simulink model "Table_airbus_v1"  (R2021b)
settings: Solver=VariableStepAuto  StartTime=0.0  StopTime=20  MaxStep=0.01  RelTol=0.01
undefined symbols (not defined in the file): X, Y, Z
libraries: sm_lib x907, fl_lib x69, nesl_utility x53, sdl_lib x10, ee_lib x7, slpidlib x6, simulink x5, simulink_extras x4
(part 1 of 18)
settings Model: Creator=Marc  LastModifiedBy=mgarc
settings SolverCC: ZeroCrossAlgorithm=Adaptive  AlgebraicLoopSolver=TrustRegion
settings DebuggingCC: IgnoredZcDiagnostic=none  SFMachineParentedDataDiag=warning  ArithmeticOperatorsInVariantConditions=warning
settings SFSimCC: CustomCodeUndefinedFunction=UseInterfaceOnly
settings ExplorerConfigSet: InternalSimMechanicsExplorerSettings="<ExplorerConfiguration><canonicalview>default</canonicalview><AnimationSetting><BasePlaybackSpeed>1.0</BasePlaybackSpeed><PlaybackSpeedFactor>1.0</PlaybackSpeedFactor></AnimationSetting><TilePanel><TileInfo><Tiles Columns=\"2\" Count=\"4\" Rows=\"2\"><Column Weight=\"0.4997\"/><Column Weight=\"0.5003\"/><Row Weight=\"0.5\"/><Row Weight=\"0.5\"/><Tile Height=\"1\" Width=\"1\" X=\"0\" Y=\"0\"/><Tile Height=\"1\" Width=\"1\" X=\"0\" Y=\"1\"/><Tile Height=\"1\" Width=\"1\" X=\"1\" Y=\"0\"/><Tile Height=\"1\" Width=\"1\" X=\"1\" Y=\"1\"/></Tiles></TileInfo><SceneInfo><SceneViewer><BGColor><R>0.60000002384185791</R><G>0.60000002384185791</G><B>0.60000002384185791</B></BGColor><Camera><DoPerspective>off</DoPerspective><Position><X>-1.24933457614355525</X><Y>-1.70068668146841429</Y><Z>0.410584900495560123</Z></Position><Center><X>-1.24933457614355525</X><Y>1.97814830626974469e-08</Y><Z>0.410584900495560123</Z></Center><Up><X>0</X><Y>-0</Y><Z>1</Z></Up><ViewLimDist>1</ViewLimDist><YLim>0.703268185423852166</YLim><XLim>1.31924547195434561</XLim></Camera></SceneViewer><SceneViewer><BGColor><R>0.60000002384185791</R><G>0.60000002384185791</G><B>0.60000002384185791</B></BGColor><Camera><DoPerspective>off</DoPerspective><Position><X>-1.24933457614355525</X><Y>4.88032186884979069e-09</Y><Z>2.2537451526153367</Z></Position><Center><X>-1.24933457614355525</X><Y>4.88032186884979069e-09</Y><Z>0.410584900495560179</Z></Center><Up><X>0</X><Y>1</Y><Z>-0</Z></Up><ViewLimDist>1</ViewLimDist><YLim>0.703268185423852166</YLim><XLim>1.31924547195434561</XLim></Camera></SceneViewer><SceneViewer><BGColor><R>0.60000002384185791</R><G>0.60000002384185791</G><B>0.60000002384185791</B></BGColor><Camera><DoPerspective>off</DoPerspective><Position><X>0.330264279532568983</X><Y>4.88032181333863946e-09</Y><Z>0.410584900495559957</Z></Position><Center><X>-1.2493346738951725</X><Y>4.88032181333863946e-09</Y><Z>0.410584900495559957</Z></Center><Up><X>-0</X><Y>0</Y><Z>1</Z></Up><ViewLimDist>1</ViewLimDist><YLim>0.415614598393440282</YLim><XLim>0.780615709394705148</XLim></Camera></SceneViewer><SceneViewer><BGColor><R>0.60000002384185791</R><G>0.60000002384185791</G><B>0.60000002384185791</B></BGColor><Camera><DoPerspective>off</DoPerspective><Position><X>-0.231613369317086537</X><Y>-0.977872883847284546</Y><Z>1.37865497927362801</Z></Position><Center><X>-1.1321755767731061</X><Y>-0.0773106763912649875</Y><Z>0.47809277181760812</Z></Center><Up><X>-0.408248290463863073</X><Y>0.408248290463863073</Y><Z>0.816496580927726145</Z></Up><ViewLimDist>1</ViewLimDist><YLim>1.00376938045024877</YLim><XLim>1.88529986679414407</XLim></Camera></SceneViewer></SceneInfo></TilePanel><MechEditorPanel><Cameras/><GfxPanelCameraMap/><VideoCreator><PlaybackSpeedRatio>1.0</PlaybackSpeedRatio><FrameRate>30</FrameRate><VideoFormat>Motion JPEG AVI</VideoFormat><FrameSize>auto</FrameSize></VideoCreator></MechEditorPanel></ExplorerConfiguration>"

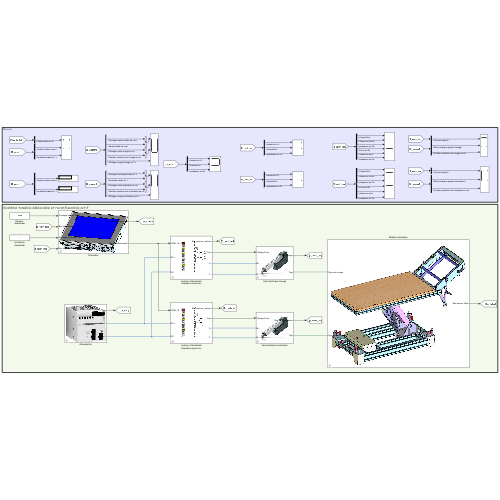
[thumbnail: Simulink's stored preview of the top-level diagram]
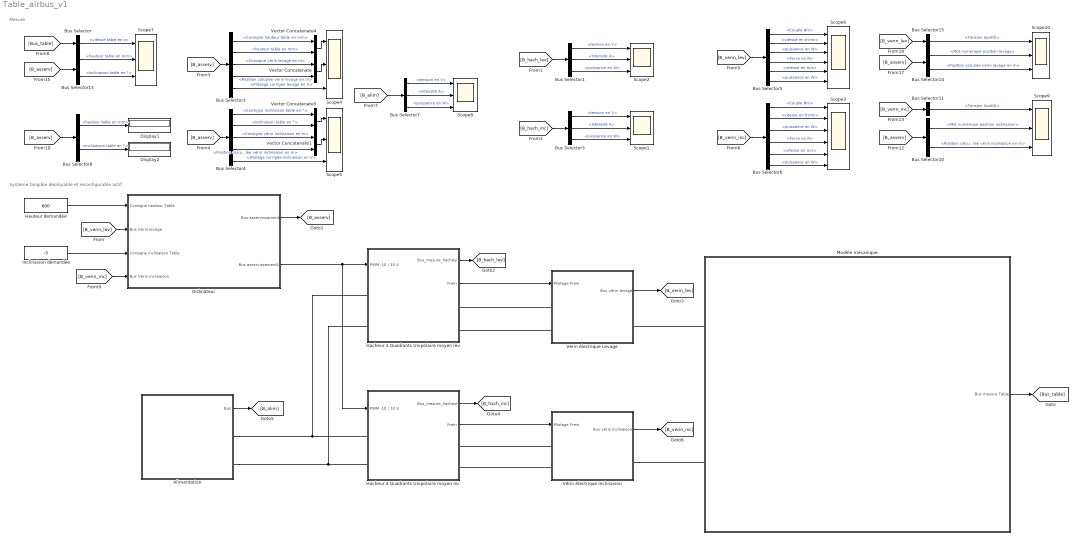
== system Table_airbus_v1 ==
  note: Mesure
  note: Système tangible déployable et reconfigurable actif
  Alimentation : Subsystem  mask{Ualim=36, Ralim=0.5}
      mask prompts: Ualim "Tension d'alimentation en V"; Ralim "Résistance interne alimentation en ohm"
      mask DialogControl ParameterGroupVar Prompt: Paramètres alimentation
      mask Display: image('alimentation.png')
  Bus Selector : BusSelector  OutputSignals=vitesse table en z
  Bus Selector1 : BusSelector  OutputSignals=tension en V,Intensité A,puissance en W
  Bus Selector10 : BusSelector  OutputSignals=Mot numérique position inclinaison,Position calculée vérin inclinaison en m
  Bus Selector11 : BusSelector  OutputSignals=Tension Upot(t)
  Bus Selector13 : BusSelector  OutputSignals=hauteur table en mm,Inclinaison table en °
  Bus Selector14 : BusSelector  OutputSignals=Mot numérique position levage,Position calculée vérin levage en m
  Bus Selector15 : BusSelector  OutputSignals=Tension Upot(t)
  Bus Selector2 : BusSelector  OutputSignals=Consigne hauteur table en mm,hauteur table en mm,Consigne vérin levage en m,Position calculée vérin levage en m,Pilotage corrigée levage en V
  Bus Selector3 : BusSelector  OutputSignals=tension en V,Intensité A,puissance en W
  Bus Selector4 : BusSelector  OutputSignals=Consigne inclinaison table en °,Inclinaison table en °,Consigne vérin inclinaison en m,Position calculée vérin inclinaison en m,Pilotage corrigée inclinaison en V
  Bus Selector5 : BusSelector  OutputSignals=Bus meca moteur.Couple Nm,Bus meca moteur.vitesse en tr/mn,Bus meca moteur.puissance en W,Bus vis écrou.Force en N,Bus vis écrou.vitesse en m/s,Bus vis écrou.puissance en W
  Bus Selector6 : BusSelector  OutputSignals=Bus meca moteur.Couple Nm,Bus meca moteur.vitesse en tr/mn,Bus meca moteur.puissance en W,Bus vis écrou.Force en N,Bus vis écrou.vitesse en m/s,Bus vis écrou.puissance en W
  Bus Selector7 : BusSelector  OutputSignals=tension en V,Intensité A,puissance en W
  Bus Selector8 : BusSelector  OutputSignals=hauteur table en mm,Inclinaison table en °
  Display1 : Display
  Display2 : Display
  Hacheur 4 Quadrants Unipolaire moyen Inc : Subsystem  mask{Rds=0.2, Rd=0.1, Vd=0.65, kpn=4, kin=1, kdn=0, Imax=8, Kpi=0.8, Kii=0, Kdi=0}
      mask prompts: Rds "Résistance drain source Mosfet en ohm"; Rd "Résistance diode source drain en ohm"; Vd "Tension de seuil diode source drain en volt"; kpn "Gain proportionnel"; kin "Gain intégral"; kdn "Gain dérivée"; Imax "Limitation d'intensité en A"; Kpi "Gain proportionnel"; Kii "Gain intégral"; Kdi "Gain dérivée"
      mask DialogControl ParameterGroupVar Prompt: Paramétrages carte d'axe
      mask DialogControl Container4 Prompt: Hacheur
      mask DialogControl Container5 Prompt: Régulation Vitesse
      mask DialogControl Container7 Prompt: Régulation d'intensité
      mask Display: image('BKH-KL2532.jpg')
  Hacheur 4 Quadrants Unipolaire moyen lev : Subsystem  mask{Rds=0.2, Rd=0.1, Vd=0.65, kpn=4, kin=1, kdn=0, Imax=8, Kpi=0.8, Kii=0, Kdi=0}
      mask prompts: Rds "Résistance drain source Mosfet en ohm"; Rd "Résistance diode source drain en ohm"; Vd "Tension de seuil diode source drain en volt"; kpn "Gain proportionnel"; kin "Gain intégral"; kdn "Gain dérivée"; Imax "Limitation d'intensité en A"; Kpi "Gain proportionnel"; Kii "Gain intégral"; Kdi "Gain dérivée"
      mask DialogControl ParameterGroupVar Prompt: Paramétrages carte d'axe
      mask DialogControl Container4 Prompt: Hacheur
      mask DialogControl Container5 Prompt: Régulation Vitesse
      mask DialogControl Container7 Prompt: Régulation d'intensité
      mask Display: image('BKH-KL2532.jpg')
  Hauteur demandée : Constant  Value=600
  Inclinaison demandée : Constant  Value=-5
  Modèle mécanique : Subsystem  mask{Fsec_Lev=20, fv_Lev=100, Fsec_Inc=20, fv_Inc=100, Mt=70}
      mask prompts: Fsec_Lev "Frottement sec en N"; fv_Lev "Coefficient de frottement visqueux en N/(m/s)"; Fsec_Inc "Frottement sec en N"; fv_Inc "Coefficient de frottement visqueux en N/(m/s)"; Mt "Masse supplémentaire en kg"
      mask DialogControl Container4 Prompt: Levage
      mask DialogControl Container1 Prompt: Inclinaison
      mask DialogControl Container8 Prompt: Masse transportée
      mask Display: image('table3d.png')
  Ordinateur : Subsystem  mask{kp_lev=10, ki_lev=0.001, kd_lev=0, kp_inc=4, ki_inc=0.001, kd_inc=0, ordre3=on, pos_lev_max=600, pos_lev_min=250, N=16}
      mask prompts: kp_lev "Coefficient proportionnel"; ki_lev "Coefficient intégral"; kd_lev "Coefficient dérivé"; kp_inc "Coefficient proportionnel"; ki_inc "Coefficient intégral"; kd_inc "Coefficient dérivé"; ordre3 "Interpolation d'ordre 3"; pos_lev_max "Hauteur maximale table en mm"; pos_lev_min "Hauteur minimale table en mm"; N "Nombre de bits du CAN (bit de signe compris)"
      mask DialogControl Container16 Prompt: Paramétrages unité de contrôle
      mask DialogControl Container30 Prompt: Configuration utilisateur
      mask DialogControl Container25 Prompt: Correcteur PID du vérin de levage
      mask DialogControl Container25_copy Prompt: Correcteur PID du vérin d'inclinaison
      mask DialogControl Container29 Prompt: Divers
      mask DialogControl Container28 Prompt: Levage
      mask DialogControl Container22 Prompt: Convertisseur analogique numérique
      mask Display: image('IHM2.png')
  Scope{1..2,4..5,7..10} (8 alike) : Scope  NumInputPorts=3
  Scope3 : Scope  NumInputPorts=6
  Scope6 : Scope  NumInputPorts=6
  Vector Concatenate{,1,4..5} (4 alike) : Concatenate
  Vérin électrique Inclinaison : Subsystem  mask{kt=0.05555, R=0.53333, L=1600, I0=1.1, U0=24, Jm=32e-5, ratio_epi=15.44, rend_epi=80, ratio_red=(58*37)/(45*16), rend_red=80, pas_vis=8, Landa=13, Alpha=14.5, fv=0.08, Pmax=150, P=10}
      mask prompts: kt "Constante de couple en N.m/A"; R "Résistance moteur en Ω"; L "Inductance moteur en µH"; I0 "Intensité consommée à vide en A"; U0 "Tension nominale moteur en V"; Jm "Inertie moteur en kg.m²"; ratio_epi "Rapport de réduction réducteur"; rend_epi "Rendement réducteur en %"; ratio_red "Rapport de réduction réducteur"; rend_red "Rendement réducteur en %"; pas_vis "Pas de vis en mm"; Landa "Angle d'attaque λ en °"; Alpha "Demi-angle de filetage acmé α en °"; fv "Coefficient de friction"; Pmax "Position maximale mesurée en mm"; P "Valeur maximale du potentiomètre en  kΩ"
      mask DialogControl ParameterGroupVar Prompt: Paramétrages du vérin électrique
      mask DialogControl Container4 Prompt: Moteur à courant continu
      mask DialogControl Container6 Prompt: Réducteur épicycloïdal
      mask DialogControl Container8 Prompt: Réducteur simple
      mask DialogControl Container10 Prompt: Transmission vis écrou
      mask DialogControl Container11 Prompt: Potentiomètre de recopie
      mask Display: image('linak.jpg')
  Vérin électrique Levage : Subsystem  mask{kt=0.05555, R=0.53333, L=1600, I0=1.1, U0=24, Jm=32e-5, ratio_epi=15.44, rend_epi=80, ratio_red=(58*37)/(45*16), rend_red=80, pas_vis=8, Landa=13, Alpha=14.5, fv=0.08, Pmax=150, P=10}
      mask prompts: kt "Constante de couple en N.m/A"; R "Résistance moteur en Ω"; L "Inductance moteur en µH"; I0 "Intensité consommée à vide en A"; U0 "Tension nominale moteur en V"; Jm "Inertie moteur en kg.m²"; ratio_epi "Rapport de réduction réducteur"; rend_epi "Rendement réducteur en %"; ratio_red "Rapport de réduction réducteur"; rend_red "Rendement réducteur en %"; pas_vis "Pas de vis en mm"; Landa "Angle d'attaque λ en °"; Alpha "Demi-angle de filetage acmé α en °"; fv "Coefficient de friction"; Pmax "Position maximale mesurée en mm"; P "Valeur maximale du potentiomètre en  kΩ"
      mask DialogControl ParameterGroupVar Prompt: Paramétrages du vérin électrique
      mask DialogControl Container4 Prompt: Moteur à courant continu
      mask DialogControl Container6 Prompt: Réducteur épicycloïdal
      mask DialogControl Container8 Prompt: Réducteur simple
      mask DialogControl Container10 Prompt: Transmission vis écrou
      mask DialogControl Container11 Prompt: Potentiomètre de recopie
      mask Display: image('linak.jpg')
  wires:
  Alimentation/1(Bus) -> [B_alim]
  Vérin électrique Levage/1(Bus vérin levage) -> [B_verin_lev]
  Inclinaison demandée/1 -> Ordinateur/3(Consigne inclinaison Table)
  Vérin électrique Inclinaison/1(Bus vérin Inclinaison) -> [B_verin_inc]
  Hacheur 4 Quadrants Unipolaire moyen Inc/1(Bus_mesure_hacheur) -> [B_hach_inc]
  Hacheur 4 Quadrants Unipolaire moyen lev/1(Bus_mesure_hacheur) -> [B_hach_lev]
  Hauteur demandée/1 -> Ordinateur/1(Consigne hauteur Table)
  [B_verin_lev] -> Ordinateur/2(Bus Vérin levage)
  Modèle mécanique/1(Bus mesure Table) -> [Bus_table]
  Bus Selector1/1 -> Scope2/1  "<tension en V>"
  Bus Selector1/2 -> Scope2/2  "<Intensité A>"
  [B_asserv] -> Bus Selector2/1
  Bus Selector2/1 -> Vector Concatenate4/1  "<Consigne hauteur table en mm>"
  Bus Selector2/3 -> Vector Concatenate/1  "<Consigne vérin levage en m>"
  Bus Selector2/4 -> Vector Concatenate/2  "<Position calculée vérin levage en m>"
  Bus Selector2/5 -> Scope4/3  "<Pilotage corrigée levage en V>"
  [B_hach_lev] -> Bus Selector1/1
  Bus Selector1/3 -> Scope2/3  "<puissance en W>"
  Bus Selector3/3 -> Scope1/3  "<puissance en W>"
  [B_hach_inc] -> Bus Selector3/1
  Bus Selector3/2 -> Scope1/2  "<Intensité A>"
  Bus Selector3/1 -> Scope1/1  "<tension en V>"
  Bus Selector4/5 -> Scope5/3  "<Pilotage corrigée inclinaison en V>"
  Bus Selector4/4 -> Vector Concatenate1/2  "<Position calculée vérin inclinaison en m>"
  Bus Selector4/3 -> Vector Concatenate1/1  "<Consigne vérin inclinaison en m>"
  Bus Selector4/1 -> Vector Concatenate5/1  "<Consigne inclinaison table en °>"
  [B_asserv] -> Bus Selector4/1
  Bus Selector5/3 -> Scope6/3  "<puissance en W>"
  [B_verin_lev] -> Bus Selector5/1
  Bus Selector5/2 -> Scope6/2  "<vitesse en tr/mn>"
  Bus Selector5/1 -> Scope6/1  "<Couple Nm>"
  Bus Selector5/4 -> Scope6/4  "<Force en N>"
  Bus Selector5/5 -> Scope6/5  "<vitesse en m/s>"
  Bus Selector5/6 -> Scope6/6  "<puissance en W>"
  Bus Selector6/6 -> Scope3/6  "<puissance en W>"
  Bus Selector6/5 -> Scope3/5  "<vitesse en m/s>"
  Bus Selector6/4 -> Scope3/4  "<Force en N>"
  Bus Selector6/1 -> Scope3/1  "<Couple Nm>"
  Bus Selector6/2 -> Scope3/2  "<vitesse en tr/mn>"
  [B_verin_inc] -> Bus Selector6/1
  Bus Selector6/3 -> Scope3/3  "<puissance en W>"
  Bus Selector7/3 -> Scope8/3  "<puissance en W>"
  [B_alim] -> Bus Selector7/1
  Bus Selector7/2 -> Scope8/2  "<Intensité A>"
  Bus Selector7/1 -> Scope8/1  "<tension en V>"
  Vector Concatenate/1 -> Scope4/2
  Vector Concatenate1/1 -> Scope5/2
  [B_verin_inc] -> Ordinateur/4(Bus Vérin inclinaison)
  [B_asserv] -> Bus Selector10/1
  Bus Selector10/1 -> Scope9/2  "<Mot numérique position inclinaison>"
  [B_verin_inc] -> Bus Selector11/1
  Bus Selector11/1 -> Scope9/1  "<Tension Upot(t)>"
  Bus Selector10/2 -> Scope9/3  "<Position calculée vérin inclinaison en m>"
  Ordinateur/2(Bus asservissement1) -> Hacheur 4 Quadrants Unipolaire moyen Inc/1("PWM -10 / 10 V "), Hacheur 4 Quadrants Unipolaire moyen lev/1("PWM -10 / 10 V ")
  Ordinateur/1(Bus asservissement) -> [B_asserv]
  Bus Selector8/2 -> Display2/1  "<Inclinaison table en °>"
  [B_asserv] -> Bus Selector8/1
  Bus Selector/1 -> Scope7/1  "<vitesse table en z>"
  [Bus_table] -> Bus Selector/1
  Bus Selector13/1 -> Scope7/2  "<hauteur table en mm>"
  Bus Selector8/1 -> Display1/1  "<hauteur table en mm>"
  Bus Selector13/2 -> Scope7/3  "<Inclinaison table en °>"
  [B_asserv] -> Bus Selector13/1
  Bus Selector14/2 -> Scope10/3  "<Position calculée vérin levage en m>"
  [B_verin_lev] -> Bus Selector15/1
  Bus Selector15/1 -> Scope10/1  "<Tension Upot(t)>"
  Bus Selector14/1 -> Scope10/2  "<Mot numérique position levage>"
  [B_asserv] -> Bus Selector14/1
  Hacheur 4 Quadrants Unipolaire moyen Inc/2(Frein) -> Vérin électrique Inclinaison/1(Pilotage Frein)
  Hacheur 4 Quadrants Unipolaire moyen lev/2(Frein) -> Vérin électrique Levage/1(Pilotage Frein)
  Bus Selector2/2 -> Vector Concatenate4/2  "<hauteur table en mm>"
  Vector Concatenate4/1 -> Scope4/1
  Vector Concatenate5/1 -> Scope5/1
  Bus Selector4/2 -> Vector Concatenate5/2  "<Inclinaison table en °>"
  connections:
  Alimentation/RConn2 -- Hacheur 4 Quadrants Unipolaire moyen Inc/LConn2 -- Hacheur 4 Quadrants Unipolaire moyen lev/LConn2
  Alimentation/RConn1 -- Hacheur 4 Quadrants Unipolaire moyen Inc/LConn1 -- Hacheur 4 Quadrants Unipolaire moyen lev/LConn1
  Vérin électrique Inclinaison/LConn2 -- Hacheur 4 Quadrants Unipolaire moyen Inc/RConn2
  Vérin électrique Inclinaison/LConn1 -- Hacheur 4 Quadrants Unipolaire moyen Inc/RConn1
  Modèle mécanique/LConn1 -- Vérin électrique Levage/RConn1
  Vérin électrique Levage/LConn1 -- Hacheur 4 Quadrants Unipolaire moyen lev/RConn1
  Vérin électrique Levage/LConn2 -- Hacheur 4 Quadrants Unipolaire moyen lev/RConn2
  Vérin électrique Inclinaison/RConn1 -- Modèle mécanique/LConn2

== system Table_airbus_v1/Alimentation ==
  Capteur électrique alim : Subsystem
  Constant3 : Constant  Value=Ualim
  Controlled Voltage Source1 : fl_lib/Electrical/Electrical Sources/Controlled Voltage Source
  Electrical Reference4 : fl_lib/Electrical/Electrical Elements/Electrical Reference
  Resistor : fl_lib/Electrical/Electrical Elements/Resistor  R=Ralim Ohm  i_specify=off  i_priority=None  i=0 A  i_nominal_specify=off  i_nominal_unit=A  i_nominal_value=1  v_specify=off  v_priority=None  v=0 V  v_nominal_specify=off  v_nominal_unit=V  v_nominal_value=1
  Simulink-PS Converter1 : nesl_utility/Simulink-PS Converter  PhysicalDomain=network_engine_domain  SubClassName=ps_input  LeftPortType=input  RightPortType=output  PseudoPeriodic=off  Frequencies=[]  NoiseDistribution=none  NoiseParameters=[]  Unit=V  AffineConversion=off  FilteringAndDerivatives=zero  SimscapeFilterOrder=1  InputFilterTimeConstant=0.001  UdotUserProvided=1
      settings: SourceProductBaseCode=PW,SS
  Solver Configuration : nesl_utility/Solver Configuration  PhysicalDomain=network_engine_domain  SubClassName=solver  LeftPortType=input  RightPortType=generic  Tones=[]  Harmonics=[]  SimulateNoise=off  Profile=off  UseLocalSampling=off  EnableSwitchedLinearOptims=on  FrequencyDomain=off  UseCCode=off  RelTol=0.001  AbsTol=1e-06  MinStep=1e-09  ToWorkspace=off  RevertToSquareIcSolve=off  NumHomotopyIterations=100  PhasorMode=off  PhasorModeNumHarmonics=1  DoDC=off  ResidualTolerance=1e-09  UseLocalSolver=off  LocalSolverChoice=NE_TRAPEZOIDAL_ADVANCER  LocalSolverSampleTime=0.001  DoFixedCost=off  MaxNonlinIter=3  MaxModeIter=2  ComputeImpulses=off  ImpulseIterations=2  LinearAlgebra=Sparse  EquationFormulation=NE_TIME_EF  DelaysMemoryBudget=1024  AutomaticFiltering=on  FilteringTimeConstant=0.001  PartitionStorageMethod=AS_NEEDED  PartitionMemoryBudget=1024  PartitionMethod=FAST
      settings: SourceProductBaseCode=PW,SS
  Alim + : PMIOPort  Side=Right
  Alim - : PMIOPort  Port=2  Side=Right
  Bus : Outport  VectorParamsAs1DForOutWhenUnconnected=off
  wires:
  Constant3/1 -> Simulink-PS Converter1/1
  Capteur électrique alim/1(Bus) -> Bus/1
  connections:
  Electrical Reference4/LConn1 -- Capteur électrique alim/LConn2 -- Controlled Voltage Source1/RConn2 -- Solver Configuration/RConn1
  Simulink-PS Converter1/RConn1 -- Controlled Voltage Source1/RConn1
  Resistor/RConn1 -- Capteur électrique alim/LConn1
  Alim -/RConn1 -- Capteur électrique alim/RConn2
  Alim +/RConn1 -- Capteur électrique alim/RConn1
  Controlled Voltage Source1/LConn1 -- Resistor/LConn1

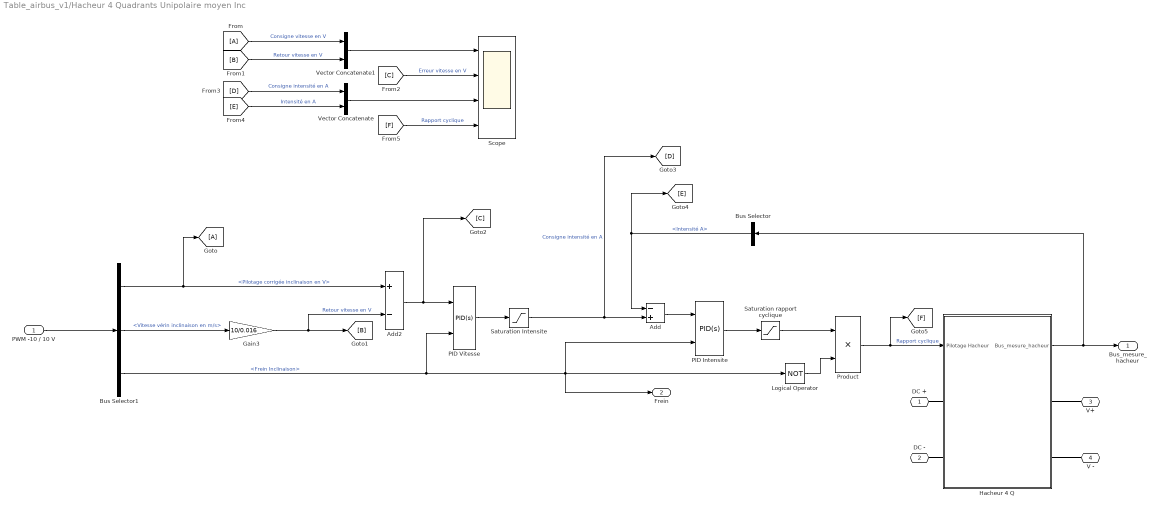
== system Table_airbus_v1/Hacheur 4 Quadrants Unipolaire moyen Inc ==
  "PWM -10 / 10 V " : Inport
  Add : Sum  Inputs=-+
  Add2 : Sum  Inputs=+-
  Bus Selector : BusSelector  OutputSignals=Intensité A
  Bus Selector1 : BusSelector  OutputSignals=Pilotage corrigée inclinaison en V,Vitesse vérin inclinaison en m/s,Frein Inclinaison
  Gain3 : Gain  Gain=10/0.016
  Hacheur 4 Q : Subsystem
  Logical Operator : Logic  Operator=NOT  AllPortsSameDT=off  OutDataTypeStr=boolean
  PID Intensite : slpidlib/PID Controller  Controller=PID  Form=Parallel  TimeDomain=Continuous-time  UseExternalTs=off  SampleTime=-1  IntegratorMethod=Forward Euler  FilterMethod=Forward Euler  ControllerParametersSource=internal  P=Kpi  I=Kii  D=Kdi  UseFilter=on  N=100  TunerSelectOption=Transfer Function Based (PID Tuner App)  InitialConditionSource=internal  InitialConditionForIntegrator=0  InitialConditionForFilter=0  DifferentiatorICPrevScaledInput=0  ExternalReset=level  TrackingMode=off  Kt=1  LimitOutput=off  SatLimitsSource=internal  UpperSaturationLimit=inf  LowerSaturationLimit=-inf  LinearizeAsGain=off  AntiWindupMode=none  Kb=1  POutMin=[]  POutMax=[]  IOutMin=[]  IOutMax=[]  DOutMin=[]  DOutMax=[]  NOutMin=[]  NOutMax=[]  SumOutMin=[]  SumOutMax=[]  SaturationOutMin=[]  SaturationOutMax=[]  PParamMin=[]  PParamMax=[]  IParamMin=[]  IParamMax=[]  DParamMin=[]  DParamMax=[]  NParamMin=[]  NParamMax=[]  KbParamMin=[]  KbParamMax=[]  KtParamMin=[]  KtParamMax=[]  KbOutMin=[]  KbOutMax=[]  KtOutMin=[]  KtOutMax=[]  IntegratorOutMin=[]  IntegratorOutMax=[]  FilterOutMin=[]  FilterOutMax=[]  SumI1OutMin=[]  SumI1OutMax=[]  SumI2OutMin=[]  SumI2OutMax=[]  SumI3OutMin=[]  SumI3OutMax=[]  SumI4OutMin=[]  SumI4OutMax=[]  SumDOutMin=[]  SumDOutMax=[]  DifferentiatorOutMin=[]  DifferentiatorOutMax=[]  FilterDiffOutCoefMin=[]  FilterDiffOutCoefMax=[]  ReciprocalOutMin=[]  ReciprocalOutMax=[]  SumDenOutMin=[]  SumDenOutMax=[]  SumNumOutMin=[]  SumNumOutMax=[]  DivideOutMin=[]  DivideOutMax=[]  UdiffTsProdOutMin=[]  UdiffTsProdOutMax=[]  NTsProdOutMin=[]  NTsProdOutMax=[]  UintegralTsProdOutMin=[]  UintegralTsProdOutMax=[]  UngainTsProdOutMin=[]  UngainTsProdOutMax=[]  IntegratorContinuousStateAttributes=''  IntegratorStateMustResolveToSignalObject=off  IntegratorRTWStateStorageClass=Auto  FilterContinuousStateAttributes=''  FilterStateMustResolveToSignalObject=off  FilterRTWStateStorageClass=Auto  ParallelPVariant=InternalParameters  IdealPVariant=Disabled  IVariant=InternalParameters  DVariant=InternalParameters  IntegratorVariant=Continuous  SatVariant=Disabled  AWVariant=Passthrough  PCopyVariant=Disabled  TRVariant=Disabled  FdbkBlocksVariant=Forward  IdealPFdbkVariant=Disabled  SatFdbkVariant=Disabled  DerivativeFilterVariant=ContFilter  NVariant=InternalParameters  NCopyVariant=Disabled  FilterICVariant=InternalICsFilter  IntegratorICVariant=InternalICs  ExternalResetVariant=ExternalReset  TRSumVariant=Passthrough  SumFdbkVariant=Disabled  SumVariant=Sum_PID  TsampFilterVariant=InternalTs  TsampNgainVariant=Passthrough  TsampIntegralVariant=Passthrough  ExternalSaturationOutDataTypeStr=Inherit: Same as second input
  PID Vitesse : slpidlib/PID Controller  Controller=PID  Form=Parallel  TimeDomain=Continuous-time  UseExternalTs=off  SampleTime=-1  IntegratorMethod=Forward Euler  FilterMethod=Forward Euler  ControllerParametersSource=internal  P=kpn  I=kin  D=kdn  UseFilter=on  N=100  TunerSelectOption=Transfer Function Based (PID Tuner App)  InitialConditionSource=internal  InitialConditionForIntegrator=0  InitialConditionForFilter=0  DifferentiatorICPrevScaledInput=0  ExternalReset=level  TrackingMode=off  Kt=1  LimitOutput=off  SatLimitsSource=internal  UpperSaturationLimit=inf  LowerSaturationLimit=-inf  LinearizeAsGain=on  AntiWindupMode=none  Kb=1  POutMin=[]  POutMax=[]  IOutMin=[]  IOutMax=[]  DOutMin=[]  DOutMax=[]  NOutMin=[]  NOutMax=[]  SumOutMin=[]  SumOutMax=[]  SaturationOutMin=[]  SaturationOutMax=[]  PParamMin=[]  PParamMax=[]  IParamMin=[]  IParamMax=[]  DParamMin=[]  DParamMax=[]  NParamMin=[]  NParamMax=[]  KbParamMin=[]  KbParamMax=[]  KtParamMin=[]  KtParamMax=[]  KbOutMin=[]  KbOutMax=[]  KtOutMin=[]  KtOutMax=[]  IntegratorOutMin=[]  IntegratorOutMax=[]  FilterOutMin=[]  FilterOutMax=[]  SumI1OutMin=[]  SumI1OutMax=[]  SumI2OutMin=[]  SumI2OutMax=[]  SumI3OutMin=[]  SumI3OutMax=[]  SumI4OutMin=[]  SumI4OutMax=[]  SumDOutMin=[]  SumDOutMax=[]  DifferentiatorOutMin=[]  DifferentiatorOutMax=[]  FilterDiffOutCoefMin=[]  FilterDiffOutCoefMax=[]  ReciprocalOutMin=[]  ReciprocalOutMax=[]  SumDenOutMin=[]  SumDenOutMax=[]  SumNumOutMin=[]  SumNumOutMax=[]  DivideOutMin=[]  DivideOutMax=[]  UdiffTsProdOutMin=[]  UdiffTsProdOutMax=[]  NTsProdOutMin=[]  NTsProdOutMax=[]  UintegralTsProdOutMin=[]  UintegralTsProdOutMax=[]  UngainTsProdOutMin=[]  UngainTsProdOutMax=[]  IntegratorContinuousStateAttributes=''  IntegratorStateMustResolveToSignalObject=off  IntegratorRTWStateStorageClass=Auto  FilterContinuousStateAttributes=''  FilterStateMustResolveToSignalObject=off  FilterRTWStateStorageClass=Auto  ParallelPVariant=InternalParameters  IdealPVariant=Disabled  IVariant=InternalParameters  DVariant=InternalParameters  IntegratorVariant=Continuous  SatVariant=Disabled  AWVariant=Passthrough  PCopyVariant=Disabled  TRVariant=Disabled  FdbkBlocksVariant=Forward  IdealPFdbkVariant=Disabled  SatFdbkVariant=Disabled  DerivativeFilterVariant=ContFilter  NVariant=InternalParameters  NCopyVariant=Disabled  FilterICVariant=InternalICsFilter  IntegratorICVariant=InternalICs  ExternalResetVariant=ExternalReset  TRSumVariant=Passthrough  SumFdbkVariant=Disabled  SumVariant=Sum_PID  TsampFilterVariant=InternalTs  TsampNgainVariant=Passthrough  TsampIntegralVariant=Passthrough  ExternalSaturationOutDataTypeStr=Inherit: Same as second input
  Product : Product
  Saturation Intensite : Saturate  UpperLimit=Imax  LowerLimit=-Imax  LinearizeAsGain=off
  Saturation rapport cyclique : Saturate  UpperLimit=1  LowerLimit=-1  LinearizeAsGain=off
  Scope : Scope  NumInputPorts=4
  Vector Concatenate : Concatenate
  Vector Concatenate1 : Concatenate
  DC + : PMIOPort  Side=Left
  DC - : PMIOPort  Port=2  Side=Left
  V+ : PMIOPort  Port=3  Side=Right
  V - : PMIOPort  Port=4  Side=Right
  Bus_mesure_hacheur : Outport  VectorParamsAs1DForOutWhenUnconnected=off
  Frein : Outport  Port=2  VectorParamsAs1DForOutWhenUnconnected=off
  wires:
  [F] -> Scope/4  "Rapport cyclique"
  [E] -> Vector Concatenate/2  "Intensité en A"
  [D] -> Vector Concatenate/1  "Consigne intensité en A"
  [C] -> Scope/2  "Erreur vitesse en V"
  [B] -> Vector Concatenate1/2  "Retour vitesse en V"
  [A] -> Vector Concatenate1/1  "Consigne vitesse en V"
  PID Intensite/1 -> Saturation rapport cyclique/1
  PID Vitesse/1 -> Saturation Intensite/1
  Add2/1 -> [C], PID Vitesse/1
  Product/1 -> Hacheur 4 Q/1(Pilotage Hacheur), [F]  "Rapport cyclique"
  Vector Concatenate1/1 -> Scope/1
  Vector Concatenate/1 -> Scope/3
  Saturation Intensite/1 -> [D], Add/2  "Consigne intensité en A"
  Gain3/1 -> Add2/2, [B]  "Retour vitesse en V"
  Add/1 -> PID Intensite/1
  Bus Selector1/2 -> Gain3/1  "<Vitesse vérin inclinaison en m/s>"
  "PWM -10 / 10 V "/1 -> Bus Selector1/1
  Bus Selector1/1 -> [A], Add2/1  "<Pilotage corrigée inclinaison en V>"
  Bus Selector/1 -> Add/1, [E]  "<Intensité A>"
  Hacheur 4 Q/1(Bus_mesure_hacheur) -> Bus_mesure_hacheur/1, Bus Selector/1
  Saturation rapport cyclique/1 -> Product/1
  Bus Selector1/3 -> Logical Operator/1, Frein/1, PID Intensite/2, PID Vitesse/2  "<Frein Inclinaison>"
  Logical Operator/1 -> Product/2
  connections:
  Hacheur 4 Q/RConn2 -- V -/RConn1
  DC -/RConn1 -- Hacheur 4 Q/LConn2
  V+/RConn1 -- Hacheur 4 Q/RConn1
  DC +/RConn1 -- Hacheur 4 Q/LConn1

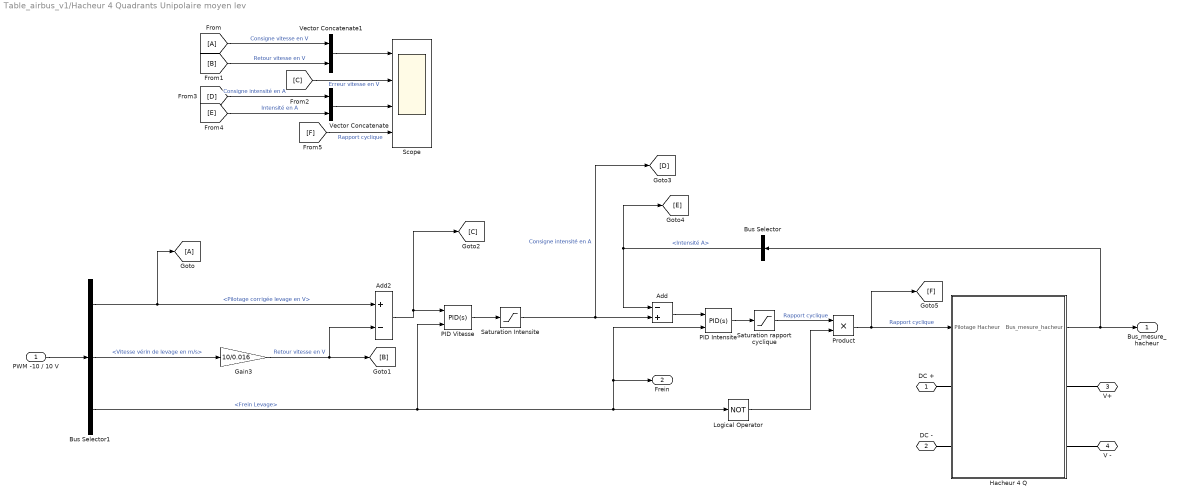
== system Table_airbus_v1/Hacheur 4 Quadrants Unipolaire moyen lev ==
  "PWM -10 / 10 V " : Inport
  Add : Sum  Inputs=-+
  Add2 : Sum  Inputs=+-
  Bus Selector : BusSelector  OutputSignals=Intensité A
  Bus Selector1 : BusSelector  OutputSignals=Pilotage corrigée levage en V,Vitesse vérin de levage en m/s,Frein Levage
  Gain3 : Gain  Gain=10/0.016
  Hacheur 4 Q : Subsystem
  Logical Operator : Logic  Operator=NOT  AllPortsSameDT=off  OutDataTypeStr=boolean
  PID Intensite : slpidlib/PID Controller  Controller=PID  Form=Parallel  TimeDomain=Continuous-time  UseExternalTs=off  SampleTime=-1  IntegratorMethod=Forward Euler  FilterMethod=Forward Euler  ControllerParametersSource=internal  P=Kpi  I=Kii  D=Kdi  UseFilter=on  N=100  TunerSelectOption=Transfer Function Based (PID Tuner App)  InitialConditionSource=internal  InitialConditionForIntegrator=0  InitialConditionForFilter=0  DifferentiatorICPrevScaledInput=0  ExternalReset=level  TrackingMode=off  Kt=1  LimitOutput=off  SatLimitsSource=internal  UpperSaturationLimit=inf  LowerSaturationLimit=-inf  LinearizeAsGain=off  AntiWindupMode=none  Kb=1  POutMin=[]  POutMax=[]  IOutMin=[]  IOutMax=[]  DOutMin=[]  DOutMax=[]  NOutMin=[]  NOutMax=[]  SumOutMin=[]  SumOutMax=[]  SaturationOutMin=[]  SaturationOutMax=[]  PParamMin=[]  PParamMax=[]  IParamMin=[]  IParamMax=[]  DParamMin=[]  DParamMax=[]  NParamMin=[]  NParamMax=[]  KbParamMin=[]  KbParamMax=[]  KtParamMin=[]  KtParamMax=[]  KbOutMin=[]  KbOutMax=[]  KtOutMin=[]  KtOutMax=[]  IntegratorOutMin=[]  IntegratorOutMax=[]  FilterOutMin=[]  FilterOutMax=[]  SumI1OutMin=[]  SumI1OutMax=[]  SumI2OutMin=[]  SumI2OutMax=[]  SumI3OutMin=[]  SumI3OutMax=[]  SumI4OutMin=[]  SumI4OutMax=[]  SumDOutMin=[]  SumDOutMax=[]  DifferentiatorOutMin=[]  DifferentiatorOutMax=[]  FilterDiffOutCoefMin=[]  FilterDiffOutCoefMax=[]  ReciprocalOutMin=[]  ReciprocalOutMax=[]  SumDenOutMin=[]  SumDenOutMax=[]  SumNumOutMin=[]  SumNumOutMax=[]  DivideOutMin=[]  DivideOutMax=[]  UdiffTsProdOutMin=[]  UdiffTsProdOutMax=[]  NTsProdOutMin=[]  NTsProdOutMax=[]  UintegralTsProdOutMin=[]  UintegralTsProdOutMax=[]  UngainTsProdOutMin=[]  UngainTsProdOutMax=[]  IntegratorContinuousStateAttributes=''  IntegratorStateMustResolveToSignalObject=off  IntegratorRTWStateStorageClass=Auto  FilterContinuousStateAttributes=''  FilterStateMustResolveToSignalObject=off  FilterRTWStateStorageClass=Auto  ParallelPVariant=InternalParameters  IdealPVariant=Disabled  IVariant=InternalParameters  DVariant=InternalParameters  IntegratorVariant=Continuous  SatVariant=Disabled  AWVariant=Passthrough  PCopyVariant=Disabled  TRVariant=Disabled  FdbkBlocksVariant=Forward  IdealPFdbkVariant=Disabled  SatFdbkVariant=Disabled  DerivativeFilterVariant=ContFilter  NVariant=InternalParameters  NCopyVariant=Disabled  FilterICVariant=InternalICsFilter  IntegratorICVariant=InternalICs  ExternalResetVariant=ExternalReset  TRSumVariant=Passthrough  SumFdbkVariant=Disabled  SumVariant=Sum_PID  TsampFilterVariant=InternalTs  TsampNgainVariant=Passthrough  TsampIntegralVariant=Passthrough  ExternalSaturationOutDataTypeStr=Inherit: Same as second input
  PID Vitesse : slpidlib/PID Controller  Controller=PID  Form=Parallel  TimeDomain=Continuous-time  UseExternalTs=off  SampleTime=-1  IntegratorMethod=Forward Euler  FilterMethod=Forward Euler  ControllerParametersSource=internal  P=kpn  I=kin  D=kdn  UseFilter=on  N=100  TunerSelectOption=Transfer Function Based (PID Tuner App)  InitialConditionSource=internal  InitialConditionForIntegrator=0  InitialConditionForFilter=0  DifferentiatorICPrevScaledInput=0  ExternalReset=level  TrackingMode=off  Kt=1  LimitOutput=off  SatLimitsSource=internal  UpperSaturationLimit=inf  LowerSaturationLimit=-inf  LinearizeAsGain=on  AntiWindupMode=none  Kb=1  POutMin=[]  POutMax=[]  IOutMin=[]  IOutMax=[]  DOutMin=[]  DOutMax=[]  NOutMin=[]  NOutMax=[]  SumOutMin=[]  SumOutMax=[]  SaturationOutMin=[]  SaturationOutMax=[]  PParamMin=[]  PParamMax=[]  IParamMin=[]  IParamMax=[]  DParamMin=[]  DParamMax=[]  NParamMin=[]  NParamMax=[]  KbParamMin=[]  KbParamMax=[]  KtParamMin=[]  KtParamMax=[]  KbOutMin=[]  KbOutMax=[]  KtOutMin=[]  KtOutMax=[]  IntegratorOutMin=[]  IntegratorOutMax=[]  FilterOutMin=[]  FilterOutMax=[]  SumI1OutMin=[]  SumI1OutMax=[]  SumI2OutMin=[]  SumI2OutMax=[]  SumI3OutMin=[]  SumI3OutMax=[]  SumI4OutMin=[]  SumI4OutMax=[]  SumDOutMin=[]  SumDOutMax=[]  DifferentiatorOutMin=[]  DifferentiatorOutMax=[]  FilterDiffOutCoefMin=[]  FilterDiffOutCoefMax=[]  ReciprocalOutMin=[]  ReciprocalOutMax=[]  SumDenOutMin=[]  SumDenOutMax=[]  SumNumOutMin=[]  SumNumOutMax=[]  DivideOutMin=[]  DivideOutMax=[]  UdiffTsProdOutMin=[]  UdiffTsProdOutMax=[]  NTsProdOutMin=[]  NTsProdOutMax=[]  UintegralTsProdOutMin=[]  UintegralTsProdOutMax=[]  UngainTsProdOutMin=[]  UngainTsProdOutMax=[]  IntegratorContinuousStateAttributes=''  IntegratorStateMustResolveToSignalObject=off  IntegratorRTWStateStorageClass=Auto  FilterContinuousStateAttributes=''  FilterStateMustResolveToSignalObject=off  FilterRTWStateStorageClass=Auto  ParallelPVariant=InternalParameters  IdealPVariant=Disabled  IVariant=InternalParameters  DVariant=InternalParameters  IntegratorVariant=Continuous  SatVariant=Disabled  AWVariant=Passthrough  PCopyVariant=Disabled  TRVariant=Disabled  FdbkBlocksVariant=Forward  IdealPFdbkVariant=Disabled  SatFdbkVariant=Disabled  DerivativeFilterVariant=ContFilter  NVariant=InternalParameters  NCopyVariant=Disabled  FilterICVariant=InternalICsFilter  IntegratorICVariant=InternalICs  ExternalResetVariant=ExternalReset  TRSumVariant=Passthrough  SumFdbkVariant=Disabled  SumVariant=Sum_PID  TsampFilterVariant=InternalTs  TsampNgainVariant=Passthrough  TsampIntegralVariant=Passthrough  ExternalSaturationOutDataTypeStr=Inherit: Same as second input
  Product : Product
  Saturation Intensite : Saturate  UpperLimit=Imax  LowerLimit=-Imax  LinearizeAsGain=off
  Saturation rapport cyclique : Saturate  UpperLimit=1  LowerLimit=-1  LinearizeAsGain=off
  Scope : Scope  NumInputPorts=4
  Vector Concatenate : Concatenate
  Vector Concatenate1 : Concatenate
  DC + : PMIOPort  Side=Left
  DC - : PMIOPort  Port=2  Side=Left
  V+ : PMIOPort  Port=3  Side=Right
  V - : PMIOPort  Port=4  Side=Right
  Bus_mesure_hacheur : Outport  VectorParamsAs1DForOutWhenUnconnected=off
  Frein : Outport  Port=2  VectorParamsAs1DForOutWhenUnconnected=off
  wires:
  Hacheur 4 Q/1(Bus_mesure_hacheur) -> Bus Selector/1, Bus_mesure_hacheur/1
  Bus Selector/1 -> [E], Add/1  "<Intensité A>"
  Bus Selector1/1 -> [A], Add2/1  "<Pilotage corrigée levage en V>"
  "PWM -10 / 10 V "/1 -> Bus Selector1/1
  Bus Selector1/2 -> Gain3/1  "<Vitesse vérin de levage en m/s>"
  Add/1 -> PID Intensite/1
  Gain3/1 -> [B], Add2/2  "Retour vitesse en V"
  Saturation Intensite/1 -> [D], Add/2  "Consigne intensité en A"
  Vector Concatenate/1 -> Scope/3
  Vector Concatenate1/1 -> Scope/1
  Product/1 -> Hacheur 4 Q/1(Pilotage Hacheur), [F]  "Rapport cyclique"
  Add2/1 -> PID Vitesse/1, [C]
  PID Vitesse/1 -> Saturation Intensite/1
  PID Intensite/1 -> Saturation rapport cyclique/1
  [A] -> Vector Concatenate1/1  "Consigne vitesse en V"
  [B] -> Vector Concatenate1/2  "Retour vitesse en V"
  [C] -> Scope/2  "Erreur vitesse en V"
  [D] -> Vector Concatenate/1  "Consigne intensité en A"
  [E] -> Vector Concatenate/2  "Intensité en A"
  [F] -> Scope/4  "Rapport cyclique"
  Bus Selector1/3 -> Frein/1, PID Intensite/2, Logical Operator/1, PID Vitesse/2  "<Frein Levage>"
  Saturation rapport cyclique/1 -> Product/1  "Rapport cyclique"
  Logical Operator/1 -> Product/2
  connections:
  DC +/RConn1 -- Hacheur 4 Q/LConn1
  V+/RConn1 -- Hacheur 4 Q/RConn1
  DC -/RConn1 -- Hacheur 4 Q/LConn2
  Hacheur 4 Q/RConn2 -- V -/RConn1

== system Table_airbus_v1/Modèle mécanique ==
  Mechanical Translational Reference : fl_lib/Mechanical/Translational Elements/Mechanical Translational Reference
  Passerelle Simscape transaltion levage : Subsystem
  Passerelle Simscape translation inclinaison : Subsystem
  Solver Configuration : nesl_utility/Solver Configuration  PhysicalDomain=network_engine_domain  SubClassName=solver  LeftPortType=input  RightPortType=generic  Tones=[]  Harmonics=[]  SimulateNoise=off  Profile=off  UseLocalSampling=off  EnableSwitchedLinearOptims=on  FrequencyDomain=off  UseCCode=off  RelTol=0.001  AbsTol=1e-06  MinStep=1e-09  ToWorkspace=off  RevertToSquareIcSolve=off  NumHomotopyIterations=100  PhasorMode=off  PhasorModeNumHarmonics=1  DoDC=off  ResidualTolerance=1e-09  UseLocalSolver=off  LocalSolverChoice=NE_BACKWARD_EULER_ADVANCER  LocalSolverSampleTime=0.001  DoFixedCost=off  MaxNonlinIter=3  MaxModeIter=2  ComputeImpulses=off  ImpulseIterations=2  LinearAlgebra=auto  EquationFormulation=NE_TIME_EF  DelaysMemoryBudget=1024  AutomaticFiltering=on  FilteringTimeConstant=0.001  PartitionStorageMethod=AS_NEEDED  PartitionMemoryBudget=1024  PartitionMethod=ROBUST
      settings: SourceProductBaseCode=PW,SS
  Table : Subsystem
  Translational Friction : fl_lib/Mechanical/Translational Elements/Translational Friction  brkwy_frc=1.25*Fsec_Lev N  brkwy_vel=0.01 m/s  Col_frc=Fsec_Lev N  visc_coef=fv_Lev N/(m/s)  v_specify=off  v_priority=None  v=0 m/s  v_nominal_specify=off  v_nominal_unit=m/s  v_nominal_value=1  f_specify=off  f_priority=None  f=0 N  f_nominal_specify=off  f_nominal_unit=N  f_nominal_value=1
      settings: SourceProductBaseCode=SS  InternalSimscapePortConfiguration="{\"Bottom\":[],\"Left\":[{\"id\":\"R\",\"label\":\"R\",\"type\":\"foundation.mechanical.translational.translational\"}],\"Right\":[{\"id\":\"C\",\"label\":\"C\",\"type\":\"foundation.mechanical.translational.translational\"}],\"Top\":[]}"
  Translational Friction2 : fl_lib/Mechanical/Translational Elements/Translational Friction  brkwy_frc=1.25*Fsec_Inc N  brkwy_vel=0.01 m/s  Col_frc=Fsec_Inc N  visc_coef=fv_Inc N/(m/s)  v_specify=off  v_priority=None  v=0 m/s  v_nominal_specify=off  v_nominal_unit=m/s  v_nominal_value=1  f_specify=off  f_priority=None  f=0 N  f_nominal_specify=off  f_nominal_unit=N  f_nominal_value=1
      settings: SourceProductBaseCode=SS  InternalSimscapePortConfiguration="{\"Bottom\":[],\"Left\":[{\"id\":\"R\",\"label\":\"R\",\"type\":\"foundation.mechanical.translational.translational\"}],\"Right\":[{\"id\":\"C\",\"label\":\"C\",\"type\":\"foundation.mechanical.translational.translational\"}],\"Top\":[]}"
  Tige verin levage : PMIOPort  Side=Left
  Tige verin inclinaison : PMIOPort  Port=2  Side=Left
  Bus mesure Table : Outport  VectorParamsAs1DForOutWhenUnconnected=off
  wires:
  Table/1(bus table) -> Bus mesure Table/1
  connections:
  Passerelle Simscape transaltion levage/RConn2 -- Table/LConn1
  Passerelle Simscape transaltion levage/RConn1 -- Table/RConn1
  Passerelle Simscape translation inclinaison/RConn1 -- Table/LConn2
  Passerelle Simscape translation inclinaison/RConn2 -- Table/RConn2
  Tige verin levage/RConn1 -- Translational Friction/LConn1 -- Passerelle Simscape transaltion levage/LConn1
  Tige verin inclinaison/RConn1 -- Translational Friction2/LConn1 -- Passerelle Simscape translation inclinaison/LConn1
  Mechanical Translational Reference/LConn1 -- Solver Configuration/RConn1 -- Translational Friction2/RConn1 -- Translational Friction/RConn1 -- Passerelle Simscape transaltion levage/LConn2 -- Passerelle Simscape translation inclinaison/LConn2
